simulink library "correlator_library"  (Simulink 6.2)
undefined symbols (not defined in the file or in its folder): BitWidthIn, BramDepth, phase_swtich_counter_width
libraries: xbsIndex_r3 x200, correlator_library x31, fft_library x11
(part 2 of 2)

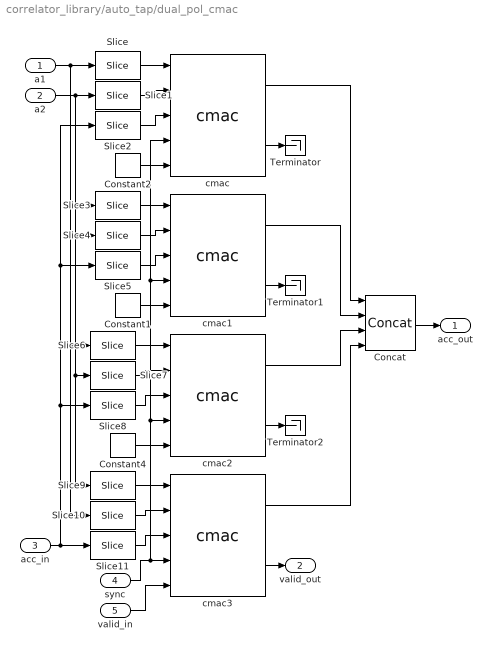
== system correlator_library/auto_tap/dual_pol_cmac ==
  a1 : Inport  Port=1  LatchInput=off
  a2 : Inport  Port=2  LatchInput=off
  acc_in : Inport  Port=3  LatchInput=off
  sync : Inport  Port=4  LatchInput=off
  valid_in : Inport  Port=5  LatchInput=off
  Concat : xbsIndex_r3/Concat  num_inputs=4  explicit_period=off  period=1  dbl_ovrd=off
  Constant1 : xbsIndex_r3/Constant  const=0  arith_type=Unsigned  n_bits=1  bin_pt=0  explicit_period=off  period=1  dbl_ovrd=off
  Constant2 : xbsIndex_r3/Constant  const=0  arith_type=Unsigned  n_bits=1  bin_pt=0  explicit_period=off  period=1  dbl_ovrd=off
  Constant4 : xbsIndex_r3/Constant  const=0  arith_type=Unsigned  n_bits=1  bin_pt=0  explicit_period=off  period=1  dbl_ovrd=off
  Slice{,1,6,9} (4 alike) : xbsIndex_r3/Slice  mode=Upper Bit Location + Width  nbits=2*BitWidthIn  bit1=0  base1=MSB of Input  bit0=0  base0=LSB of Input  boolean_output=off  explicit_period=off  period=1  dbl_ovrd=off
  Slice{3..4,7,10} (4 alike) : xbsIndex_r3/Slice  mode=Upper Bit Location + Width  nbits=2*BitWidthIn  bit1=-2*BitWidthIn  base1=MSB of Input  bit0=0  base0=LSB of Input  boolean_output=off  explicit_period=off  period=1  dbl_ovrd=off
  Slice11 : xbsIndex_r3/Slice  mode=Upper Bit Location + Width  nbits=2*BitWidthOut  bit1=-6*BitWidthOut  base1=MSB of Input  bit0=0  base0=LSB of Input  boolean_output=off  explicit_period=off  period=1  dbl_ovrd=off
  Slice2 : xbsIndex_r3/Slice  mode=Upper Bit Location + Width  nbits=2*BitWidthOut  bit1=0  base1=MSB of Input  bit0=0  base0=LSB of Input  boolean_output=off  explicit_period=off  period=1  dbl_ovrd=off
  Slice5 : xbsIndex_r3/Slice  mode=Upper Bit Location + Width  nbits=2*BitWidthOut  bit1=-2*BitWidthOut  base1=MSB of Input  bit0=0  base0=LSB of Input  boolean_output=off  explicit_period=off  period=1  dbl_ovrd=off
  Slice8 : xbsIndex_r3/Slice  mode=Upper Bit Location + Width  nbits=2*BitWidthOut  bit1=-4*BitWidthOut  base1=MSB of Input  bit0=0  base0=LSB of Input  boolean_output=off  explicit_period=off  period=1  dbl_ovrd=off
  Terminator : Terminator
  Terminator1 : Terminator
  Terminator2 : Terminator
  cmac{,1..3} (4 alike) : correlator_library/cmac  BitWidthIn=BitWidthIn  BitWidthOut=BitWidthOut  AccLen=AccLen  MultLatency=MultLatency  AddLatency=AddLatency  use_conj=on  use_mult_core=off
  acc_out : Outport
  valid_out : Outport  Port=2
  wires:
  Slice/1 -> cmac/1
  Slice1/1 -> cmac/2
  Slice2/1 -> cmac/3
  Slice3/1 -> cmac1/1
  Slice4/1 -> cmac1/2
  Slice5/1 -> cmac1/3
  Concat/1 -> acc_out/1
  Constant2/1 -> cmac/5
  cmac/2 -> Terminator/1
  Constant1/1 -> cmac1/5
  Slice6/1 -> cmac2/1
  Slice7/1 -> cmac2/2
  Slice8/1 -> cmac2/3
  Constant4/1 -> cmac2/5
  Slice9/1 -> cmac3/1
  Slice10/1 -> cmac3/2
  Slice11/1 -> cmac3/3
  valid_in/1 -> cmac3/5
  sync/1 -> cmac3/4, cmac2/4, cmac1/4, cmac/4
  cmac1/2 -> Terminator1/1
  cmac2/2 -> Terminator2/1
  cmac3/2 -> valid_out/1
  cmac/1 -> Concat/1
  cmac1/1 -> Concat/2
  cmac2/1 -> Concat/3
  cmac3/1 -> Concat/4
  a1/1 -> Slice/1, Slice3/1, Slice6/1, Slice10/1
  a2/1 -> Slice1/1, Slice4/1, Slice7/1, Slice9/1
  acc_in/1 -> Slice11/1, Slice8/1, Slice5/1, Slice2/1

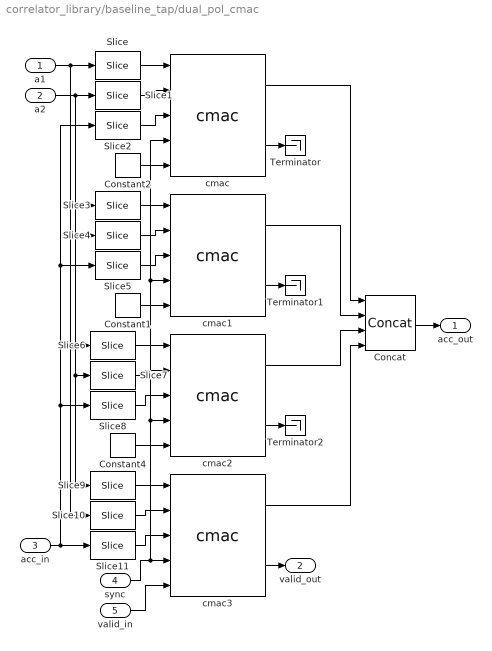
== system correlator_library/baseline_tap/dual_pol_cmac ==
  a1 : Inport  Port=1  LatchInput=off
  a2 : Inport  Port=2  LatchInput=off
  acc_in : Inport  Port=3  LatchInput=off
  sync : Inport  Port=4  LatchInput=off
  valid_in : Inport  Port=5  LatchInput=off
  Concat : xbsIndex_r3/Concat  num_inputs=4  explicit_period=off  period=1  dbl_ovrd=off
  Constant1 : xbsIndex_r3/Constant  const=0  arith_type=Unsigned  n_bits=1  bin_pt=0  explicit_period=off  period=1  dbl_ovrd=off
  Constant2 : xbsIndex_r3/Constant  const=0  arith_type=Unsigned  n_bits=1  bin_pt=0  explicit_period=off  period=1  dbl_ovrd=off
  Constant4 : xbsIndex_r3/Constant  const=0  arith_type=Unsigned  n_bits=1  bin_pt=0  explicit_period=off  period=1  dbl_ovrd=off
  Slice{,1,6,9} (4 alike) : xbsIndex_r3/Slice  mode=Upper Bit Location + Width  nbits=2*BitWidthIn  bit1=0  base1=MSB of Input  bit0=0  base0=LSB of Input  boolean_output=off  explicit_period=off  period=1  dbl_ovrd=off
  Slice{3..4,7,10} (4 alike) : xbsIndex_r3/Slice  mode=Upper Bit Location + Width  nbits=2*BitWidthIn  bit1=-2*BitWidthIn  base1=MSB of Input  bit0=0  base0=LSB of Input  boolean_output=off  explicit_period=off  period=1  dbl_ovrd=off
  Slice11 : xbsIndex_r3/Slice  mode=Upper Bit Location + Width  nbits=2*BitWidthOut  bit1=-6*BitWidthOut  base1=MSB of Input  bit0=0  base0=LSB of Input  boolean_output=off  explicit_period=off  period=1  dbl_ovrd=off
  Slice2 : xbsIndex_r3/Slice  mode=Upper Bit Location + Width  nbits=2*BitWidthOut  bit1=0  base1=MSB of Input  bit0=0  base0=LSB of Input  boolean_output=off  explicit_period=off  period=1  dbl_ovrd=off
  Slice5 : xbsIndex_r3/Slice  mode=Upper Bit Location + Width  nbits=2*BitWidthOut  bit1=-2*BitWidthOut  base1=MSB of Input  bit0=0  base0=LSB of Input  boolean_output=off  explicit_period=off  period=1  dbl_ovrd=off
  Slice8 : xbsIndex_r3/Slice  mode=Upper Bit Location + Width  nbits=2*BitWidthOut  bit1=-4*BitWidthOut  base1=MSB of Input  bit0=0  base0=LSB of Input  boolean_output=off  explicit_period=off  period=1  dbl_ovrd=off
  Terminator : Terminator
  Terminator1 : Terminator
  Terminator2 : Terminator
  cmac{,1..3} (4 alike) : correlator_library/cmac  BitWidthIn=BitWidthIn  BitWidthOut=BitWidthOut  AccLen=AccLen  MultLatency=MultLatency  AddLatency=AddLatency  use_conj=on  use_mult_core=off
  acc_out : Outport
  valid_out : Outport  Port=2
  wires:
  acc_in/1 -> Slice2/1, Slice5/1, Slice8/1, Slice11/1
  a2/1 -> Slice9/1, Slice7/1, Slice4/1, Slice1/1
  a1/1 -> Slice10/1, Slice6/1, Slice3/1, Slice/1
  cmac3/1 -> Concat/4
  cmac2/1 -> Concat/3
  cmac1/1 -> Concat/2
  cmac/1 -> Concat/1
  cmac3/2 -> valid_out/1
  cmac2/2 -> Terminator2/1
  cmac1/2 -> Terminator1/1
  sync/1 -> cmac/4, cmac1/4, cmac2/4, cmac3/4
  valid_in/1 -> cmac3/5
  Slice11/1 -> cmac3/3
  Slice10/1 -> cmac3/2
  Slice9/1 -> cmac3/1
  Constant4/1 -> cmac2/5
  Slice8/1 -> cmac2/3
  Slice7/1 -> cmac2/2
  Slice6/1 -> cmac2/1
  Constant1/1 -> cmac1/5
  cmac/2 -> Terminator/1
  Constant2/1 -> cmac/5
  Concat/1 -> acc_out/1
  Slice5/1 -> cmac1/3
  Slice4/1 -> cmac1/2
  Slice3/1 -> cmac1/1
  Slice2/1 -> cmac/3
  Slice1/1 -> cmac/2
  Slice/1 -> cmac/1

== system correlator_library/cm/cm ==
  a : Inport  Port=1  LatchInput=off
  b : Inport  Port=2  LatchInput=off
  c : Inport  Port=3  LatchInput=off
  d : Inport  Port=4  LatchInput=off
  ac : xbsIndex_r3/Mult  precision=Full  arith_type="Signed  (2's comp)"  n_bits=8  bin_pt=2  quantization=Truncate  overflow=Wrap  latency=mult_latency  explicit_period=off  period=1  en=off  dbl_ovrd=off  show_param=off  mult_type=Parallel  oversample=2  use_embedded=on  pipeline=on  use_rpm=on  placement_style=Rectangular Shape  gen_core=off
      settings: xl_area=[0, 0, 0, 0, 0, 0, 0]
  ad : xbsIndex_r3/Mult  precision=Full  arith_type="Signed  (2's comp)"  n_bits=8  bin_pt=2  quantization=Truncate  overflow=Wrap  latency=mult_latency  explicit_period=off  period=1  en=off  dbl_ovrd=off  show_param=off  mult_type=Parallel  oversample=2  use_embedded=on  pipeline=on  use_rpm=on  placement_style=Rectangular Shape  gen_core=off
      settings: xl_area=[0, 0, 0, 0, 0, 0, 0]
  bc : xbsIndex_r3/Mult  precision=Full  arith_type="Signed  (2's comp)"  n_bits=8  bin_pt=2  quantization=Truncate  overflow=Wrap  latency=mult_latency  explicit_period=off  period=1  en=off  dbl_ovrd=off  show_param=off  mult_type=Parallel  oversample=2  use_embedded=on  pipeline=on  use_rpm=on  placement_style=Rectangular Shape  gen_core=off
      settings: xl_area=[0, 0, 0, 0, 0, 0, 0]
  bd : xbsIndex_r3/Mult  precision=Full  arith_type="Signed  (2's comp)"  n_bits=8  bin_pt=2  quantization=Truncate  overflow=Wrap  latency=mult_latency  explicit_period=off  period=1  en=off  dbl_ovrd=off  show_param=off  mult_type=Parallel  oversample=2  use_embedded=on  pipeline=on  use_rpm=on  placement_style=Rectangular Shape  gen_core=off
      settings: xl_area=[0, 0, 0, 0, 0, 0, 0]
  imag_sum : xbsIndex_r3/AddSub  mode=Subtraction  precision=User Defined  arith_type=Unsigned  n_bits=n_bits  bin_pt=bin_pt  quantization="Round  (unbiased: +/- Inf)"  overflow=Wrap  latency=add_latency  explicit_period=off  period=1  use_carryin=off  use_carryout=off  en=off  dbl_ovrd=off  show_param=off  use_core=on  pipeline=off  use_rpm=on  gen_core=off
      settings: xl_area=[0, 0, 0, 0, 0, 0, 0]
  real_sum : xbsIndex_r3/AddSub  mode=Addition  precision=User Defined  arith_type=Unsigned  n_bits=n_bits  bin_pt=bin_pt  quantization="Round  (unbiased: +/- Inf)"  overflow=Wrap  latency=add_latency  explicit_period=off  period=1  use_carryin=off  use_carryout=off  en=off  dbl_ovrd=off  show_param=off  use_core=on  pipeline=off  use_rpm=on  gen_core=off
      settings: xl_area=[0, 0, 0, 0, 0, 0, 0]
  real : Outport
  imag : Outport  Port=2
  wires:
  imag_sum/1 -> imag/1
  real_sum/1 -> real/1
  d/1 -> bd/2, ad/2
  b/1 -> bd/1, bc/1
  c/1 -> ac/2, bc/2
  a/1 -> ac/1, ad/1
  ad/1 -> imag_sum/2
  bc/1 -> imag_sum/1
  bd/1 -> real_sum/2
  ac/1 -> real_sum/1

== system correlator_library/x_engine/auto_tap ==
  a_del : Inport  Port=1  LatchInput=off
  a_ndel : Inport  Port=2  LatchInput=off
  a_loop : Inport  Port=3  LatchInput=off
  a_end : Inport  Port=4  LatchInput=off
  acc_in : Inport  Port=5  LatchInput=off
  valid_in : Inport  Port=6  LatchInput=off
  sync_in : Inport  Port=7  LatchInput=off
  Delay6 : xbsIndex_r3/Delay  latency=1  reg_retiming=off  explicit_period=off  period=1  en=off  accept_only_valid=off  init_zero=on  dbl_ovrd=off  show_param=off
      settings: xl_area=[0, 0, 0, 0, 0, 0, 0]
  dual_pol_cmac : Subsystem  mask{BitWidthIn=BitWidthIn, BitWidthOut=BitWidthOut, AccLen=AccLen, MultLatency=MultLatency, AddLatency=AddLatency, use_mult_core=off}
      mask prompts: BitWidthIn "Bit Width of Sample In"; BitWidthOut "Bit Width of Sample Out"; AccLen "Accumulation Length"; MultLatency "Mult Latency"; AddLatency "Add Latency"; use_mult_core "Use Dedicated Multipliers"
      mask init: same as correlator_library/auto_tap/dual_pol_cmac
  a_del_out : Outport
  a_ndel_out : Outport  Port=2
  a_loop_out : Outport  Port=3
  a_end_out : Outport  Port=4
  acc_out : Outport  Port=5
  valid_out : Outport  Port=6
  rst_out : Outport  Port=7
  sync_out : Outport  Port=8
  wires:
  Delay6/1 -> dual_pol_cmac/4(sync)
  sync_in/1 -> sync_out/1, Delay6/1, rst_out/1
  a_del/1 -> dual_pol_cmac/1(a1), a_del_out/1
  dual_pol_cmac/1(acc_out) -> acc_out/1
  acc_in/1 -> dual_pol_cmac/3(acc_in)
  dual_pol_cmac/2(valid_out) -> valid_out/1
  valid_in/1 -> dual_pol_cmac/5(valid_in)
  a_ndel/1 -> dual_pol_cmac/2(a2), a_ndel_out/1
  a_end/1 -> a_end_out/1
  a_loop/1 -> a_loop_out/1

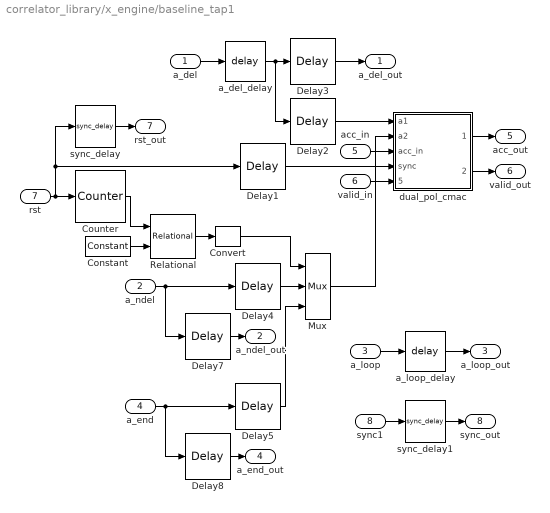
== system correlator_library/x_engine/baseline_tap1 ==
  a_del : Inport  Port=1  LatchInput=off
  a_ndel : Inport  Port=2  LatchInput=off
  a_loop : Inport  Port=3  LatchInput=off
  a_end : Inport  Port=4  LatchInput=off
  acc_in : Inport  Port=5  LatchInput=off
  valid_in : Inport  Port=6  LatchInput=off
  rst : Inport  Port=7  LatchInput=off
  sync1 : Inport  Port=8  LatchInput=off
  Constant : xbsIndex_r3/Constant  const=(AntNum - AntSep) * AccLen  equ=P=C  arith_type=Unsigned  n_bits=AntBits + BitGrowth  bin_pt=0  opselect=C  inp2=PCIN>>17  opr=+  inp1=P  carry=CIN  iostate=0  explicit_period=off  period=1  dbl_ovrd=off
  Convert : xbsIndex_r3/Convert  arith_type=Unsigned  n_bits=1  bin_pt=0  quantization=Truncate  overflow=Wrap  latency=0  explicit_period=off  period=1  dbl_ovrd=off  show_param=off  inserted_by_tool=off  pipeline=off
      settings: xl_area=[0, 0, 0, 0, 0, 0, 0]
  Counter : xbsIndex_r3/Counter  cnt_type=Count Limited  n_bits=AntBits + BitGrowth  bin_pt=0  arith_type=Unsigned  start_count=0  cnt_to=AntNum * AccLen - 1  cnt_by_val=1  operation=Up  explicit_period=off  period=1  load_pin=off  rst=on  en=off  dbl_ovrd=off  show_param=off  use_rpm=on  gen_core=off
      settings: xl_area=[0, 0, 0, 0, 0, 0, 0]
  Delay1 : xbsIndex_r3/Delay  latency=2  reg_retiming=off  explicit_period=off  period=1  en=off  accept_only_valid=off  init_zero=on  dbl_ovrd=off  show_param=off
      settings: xl_area=[0, 0, 0, 0, 0, 0, 0]
  Delay2 : xbsIndex_r3/Delay  latency=2  reg_retiming=off  explicit_period=off  period=1  en=off  accept_only_valid=off  init_zero=on  dbl_ovrd=off  show_param=off
      settings: xl_area=[0, 0, 0, 0, 0, 0, 0]
  Delay3 : xbsIndex_r3/Delay  latency=1  reg_retiming=off  explicit_period=off  period=1  en=off  accept_only_valid=off  init_zero=on  dbl_ovrd=off  show_param=off
      settings: xl_area=[0, 0, 0, 0, 0, 0, 0]
  Delay{4..5,7..8} (4 alike) : xbsIndex_r3/Delay  latency=1  reg_retiming=off  explicit_period=on  period=1  en=off  accept_only_valid=off  init_zero=on  dbl_ovrd=off  show_param=off
      settings: xl_area=[0, 0, 0, 0, 0, 0, 0]
  Mux : xbsIndex_r3/Mux  inputs=2  precision=Full  arith_type="Signed  (2's comp)"  n_bits=8  bin_pt=2  quantization=Truncate  overflow=Wrap  latency=1  explicit_period=off  period=1  en=off  dbl_ovrd=off  show_param=off  mux_type=off  use_rpm=off  gen_core=off
      settings: xl_area=[0, 0, 0, 0, 0, 0, 0]
  Relational : xbsIndex_r3/Relational  mode=a>=b  latency=1  explicit_period=off  period=1  en=off  dbl_ovrd=off  show_param=off
      settings: xl_area=[0, 0, 0, 0, 0, 0, 0]
  a_del_delay : fft_library/delay  DelayLen=AccLen
  a_loop_delay : fft_library/delay  DelayLen=AccLen - 1
  dual_pol_cmac : Subsystem  mask{BitWidthIn=BitWidthIn, BitWidthOut=BitWidthOut, AccLen=AccLen, MultLatency=MultLatency, AddLatency=AddLatency, use_mult_core=off}
      mask prompts: BitWidthIn "Bit Width of Sample In"; BitWidthOut "Bit Width of Sample Out"; AccLen "Accumulation Length"; MultLatency "Mult Latency"; AddLatency "Add Latency"; use_mult_core "Use Dedicated Multipliers"
      mask init: same as correlator_library/auto_tap/dual_pol_cmac
  sync_delay : fft_library/sync_delay  DelayLen=AccLen + 1
  sync_delay1 : fft_library/sync_delay  DelayLen=2 * AccLen
  a_del_out : Outport
  a_ndel_out : Outport  Port=2
  a_loop_out : Outport  Port=3
  a_end_out : Outport  Port=4
  acc_out : Outport  Port=5
  valid_out : Outport  Port=6
  rst_out : Outport  Port=7
  sync_out : Outport  Port=8
  wires:
  sync1/1 -> sync_delay1/1
  sync_delay1/1 -> sync_out/1
  sync_delay/1 -> rst_out/1
  Delay8/1 -> a_end_out/1
  Delay7/1 -> a_ndel_out/1
  Delay3/1 -> a_del_out/1
  a_loop_delay/1 -> a_loop_out/1
  a_loop/1 -> a_loop_delay/1
  a_end/1 -> Delay8/1, Delay5/1
  a_ndel/1 -> Delay7/1, Delay4/1
  valid_in/1 -> dual_pol_cmac/5(valid_in)
  dual_pol_cmac/2(valid_out) -> valid_out/1
  acc_in/1 -> dual_pol_cmac/3(acc_in)
  dual_pol_cmac/1(acc_out) -> acc_out/1
  a_del/1 -> a_del_delay/1
  rst/1 -> sync_delay/1, Delay1/1, Counter/1
  Delay1/1 -> dual_pol_cmac/4(sync)
  Convert/1 -> Mux/1
  Relational/1 -> Convert/1
  Constant/1 -> Relational/2
  Counter/1 -> Relational/1
  Mux/1 -> dual_pol_cmac/2(a2)
  Delay2/1 -> dual_pol_cmac/1(a1)
  a_del_delay/1 -> Delay3/1, Delay2/1
  Delay5/1 -> Mux/3
  Delay4/1 -> Mux/2

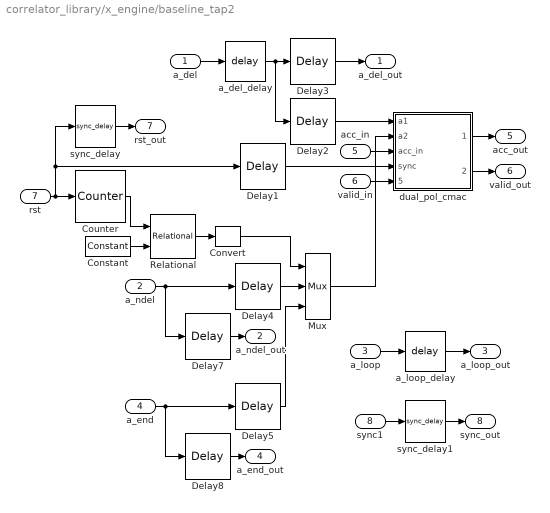
== system correlator_library/x_engine/baseline_tap2 ==
  a_del : Inport  Port=1  LatchInput=off
  a_ndel : Inport  Port=2  LatchInput=off
  a_loop : Inport  Port=3  LatchInput=off
  a_end : Inport  Port=4  LatchInput=off
  acc_in : Inport  Port=5  LatchInput=off
  valid_in : Inport  Port=6  LatchInput=off
  rst : Inport  Port=7  LatchInput=off
  sync1 : Inport  Port=8  LatchInput=off
  Constant : xbsIndex_r3/Constant  const=(AntNum - AntSep) * AccLen  equ=P=C  arith_type=Unsigned  n_bits=AntBits + BitGrowth  bin_pt=0  opselect=C  inp2=PCIN>>17  opr=+  inp1=P  carry=CIN  iostate=0  explicit_period=off  period=1  dbl_ovrd=off
  Convert : xbsIndex_r3/Convert  arith_type=Unsigned  n_bits=1  bin_pt=0  quantization=Truncate  overflow=Wrap  latency=0  explicit_period=off  period=1  dbl_ovrd=off  show_param=off  inserted_by_tool=off  pipeline=off
      settings: xl_area=[0, 0, 0, 0, 0, 0, 0]
  Counter : xbsIndex_r3/Counter  cnt_type=Count Limited  n_bits=AntBits + BitGrowth  bin_pt=0  arith_type=Unsigned  start_count=0  cnt_to=AntNum * AccLen - 1  cnt_by_val=1  operation=Up  explicit_period=off  period=1  load_pin=off  rst=on  en=off  dbl_ovrd=off  show_param=off  use_rpm=on  gen_core=off
      settings: xl_area=[0, 0, 0, 0, 0, 0, 0]
  Delay1 : xbsIndex_r3/Delay  latency=2  reg_retiming=off  explicit_period=off  period=1  en=off  accept_only_valid=off  init_zero=on  dbl_ovrd=off  show_param=off
      settings: xl_area=[0, 0, 0, 0, 0, 0, 0]
  Delay2 : xbsIndex_r3/Delay  latency=2  reg_retiming=off  explicit_period=off  period=1  en=off  accept_only_valid=off  init_zero=on  dbl_ovrd=off  show_param=off
      settings: xl_area=[0, 0, 0, 0, 0, 0, 0]
  Delay3 : xbsIndex_r3/Delay  latency=1  reg_retiming=off  explicit_period=off  period=1  en=off  accept_only_valid=off  init_zero=on  dbl_ovrd=off  show_param=off
      settings: xl_area=[0, 0, 0, 0, 0, 0, 0]
  Delay{4..5,7..8} (4 alike) : xbsIndex_r3/Delay  latency=1  reg_retiming=off  explicit_period=on  period=1  en=off  accept_only_valid=off  init_zero=on  dbl_ovrd=off  show_param=off
      settings: xl_area=[0, 0, 0, 0, 0, 0, 0]
  Mux : xbsIndex_r3/Mux  inputs=2  precision=Full  arith_type="Signed  (2's comp)"  n_bits=8  bin_pt=2  quantization=Truncate  overflow=Wrap  latency=1  explicit_period=off  period=1  en=off  dbl_ovrd=off  show_param=off  mux_type=off  use_rpm=off  gen_core=off
      settings: xl_area=[0, 0, 0, 0, 0, 0, 0]
  Relational : xbsIndex_r3/Relational  mode=a>=b  latency=1  explicit_period=off  period=1  en=off  dbl_ovrd=off  show_param=off
      settings: xl_area=[0, 0, 0, 0, 0, 0, 0]
  a_del_delay : fft_library/delay  DelayLen=AccLen
  a_loop_delay : fft_library/delay  DelayLen=AccLen - 1
  dual_pol_cmac : Subsystem  mask{BitWidthIn=BitWidthIn, BitWidthOut=BitWidthOut, AccLen=AccLen, MultLatency=MultLatency, AddLatency=AddLatency, use_mult_core=off}
      mask prompts: BitWidthIn "Bit Width of Sample In"; BitWidthOut "Bit Width of Sample Out"; AccLen "Accumulation Length"; MultLatency "Mult Latency"; AddLatency "Add Latency"; use_mult_core "Use Dedicated Multipliers"
      mask init: same as correlator_library/auto_tap/dual_pol_cmac
  sync_delay : fft_library/sync_delay  DelayLen=AccLen + 1
  sync_delay1 : fft_library/sync_delay  DelayLen=2 * AccLen
  a_del_out : Outport
  a_ndel_out : Outport  Port=2
  a_loop_out : Outport  Port=3
  a_end_out : Outport  Port=4
  acc_out : Outport  Port=5
  valid_out : Outport  Port=6
  rst_out : Outport  Port=7
  sync_out : Outport  Port=8
  wires:
  sync1/1 -> sync_delay1/1
  sync_delay1/1 -> sync_out/1
  sync_delay/1 -> rst_out/1
  Delay8/1 -> a_end_out/1
  Delay7/1 -> a_ndel_out/1
  Delay3/1 -> a_del_out/1
  a_loop_delay/1 -> a_loop_out/1
  a_loop/1 -> a_loop_delay/1
  a_end/1 -> Delay8/1, Delay5/1
  a_ndel/1 -> Delay7/1, Delay4/1
  valid_in/1 -> dual_pol_cmac/5(valid_in)
  dual_pol_cmac/2(valid_out) -> valid_out/1
  acc_in/1 -> dual_pol_cmac/3(acc_in)
  dual_pol_cmac/1(acc_out) -> acc_out/1
  a_del/1 -> a_del_delay/1
  rst/1 -> sync_delay/1, Delay1/1, Counter/1
  Delay1/1 -> dual_pol_cmac/4(sync)
  Convert/1 -> Mux/1
  Relational/1 -> Convert/1
  Constant/1 -> Relational/2
  Counter/1 -> Relational/1
  Mux/1 -> dual_pol_cmac/2(a2)
  Delay2/1 -> dual_pol_cmac/1(a1)
  a_del_delay/1 -> Delay3/1, Delay2/1
  Delay5/1 -> Mux/3
  Delay4/1 -> Mux/2

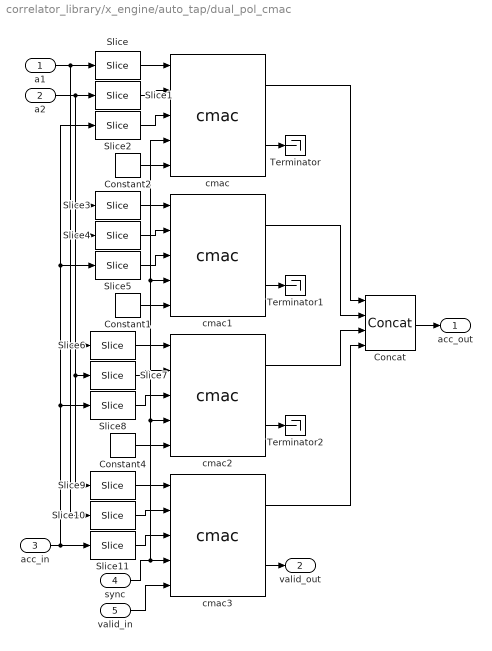
== system correlator_library/x_engine/auto_tap/dual_pol_cmac ==
  a1 : Inport  Port=1  LatchInput=off
  a2 : Inport  Port=2  LatchInput=off
  acc_in : Inport  Port=3  LatchInput=off
  sync : Inport  Port=4  LatchInput=off
  valid_in : Inport  Port=5  LatchInput=off
  Concat : xbsIndex_r3/Concat  num_inputs=4  explicit_period=off  period=1  dbl_ovrd=off
  Constant1 : xbsIndex_r3/Constant  const=0  arith_type=Unsigned  n_bits=1  bin_pt=0  explicit_period=off  period=1  dbl_ovrd=off
  Constant2 : xbsIndex_r3/Constant  const=0  arith_type=Unsigned  n_bits=1  bin_pt=0  explicit_period=off  period=1  dbl_ovrd=off
  Constant4 : xbsIndex_r3/Constant  const=0  arith_type=Unsigned  n_bits=1  bin_pt=0  explicit_period=off  period=1  dbl_ovrd=off
  Slice{,1,6,9} (4 alike) : xbsIndex_r3/Slice  mode=Upper Bit Location + Width  nbits=2*BitWidthIn  bit1=0  base1=MSB of Input  bit0=0  base0=LSB of Input  boolean_output=off  explicit_period=off  period=1  dbl_ovrd=off
  Slice{3..4,7,10} (4 alike) : xbsIndex_r3/Slice  mode=Upper Bit Location + Width  nbits=2*BitWidthIn  bit1=-2*BitWidthIn  base1=MSB of Input  bit0=0  base0=LSB of Input  boolean_output=off  explicit_period=off  period=1  dbl_ovrd=off
  Slice11 : xbsIndex_r3/Slice  mode=Upper Bit Location + Width  nbits=2*BitWidthOut  bit1=-6*BitWidthOut  base1=MSB of Input  bit0=0  base0=LSB of Input  boolean_output=off  explicit_period=off  period=1  dbl_ovrd=off
  Slice2 : xbsIndex_r3/Slice  mode=Upper Bit Location + Width  nbits=2*BitWidthOut  bit1=0  base1=MSB of Input  bit0=0  base0=LSB of Input  boolean_output=off  explicit_period=off  period=1  dbl_ovrd=off
  Slice5 : xbsIndex_r3/Slice  mode=Upper Bit Location + Width  nbits=2*BitWidthOut  bit1=-2*BitWidthOut  base1=MSB of Input  bit0=0  base0=LSB of Input  boolean_output=off  explicit_period=off  period=1  dbl_ovrd=off
  Slice8 : xbsIndex_r3/Slice  mode=Upper Bit Location + Width  nbits=2*BitWidthOut  bit1=-4*BitWidthOut  base1=MSB of Input  bit0=0  base0=LSB of Input  boolean_output=off  explicit_period=off  period=1  dbl_ovrd=off
  Terminator : Terminator
  Terminator1 : Terminator
  Terminator2 : Terminator
  cmac{,1..3} (4 alike) : correlator_library/cmac  BitWidthIn=BitWidthIn  BitWidthOut=BitWidthOut  AccLen=AccLen  MultLatency=MultLatency  AddLatency=AddLatency  use_conj=on  use_mult_core=off
  acc_out : Outport
  valid_out : Outport  Port=2
  wires:
  acc_in/1 -> Slice2/1, Slice5/1, Slice8/1, Slice11/1
  a2/1 -> Slice9/1, Slice7/1, Slice4/1, Slice1/1
  a1/1 -> Slice10/1, Slice6/1, Slice3/1, Slice/1
  cmac3/1 -> Concat/4
  cmac2/1 -> Concat/3
  cmac1/1 -> Concat/2
  cmac/1 -> Concat/1
  cmac3/2 -> valid_out/1
  cmac2/2 -> Terminator2/1
  cmac1/2 -> Terminator1/1
  sync/1 -> cmac/4, cmac1/4, cmac2/4, cmac3/4
  valid_in/1 -> cmac3/5
  Slice11/1 -> cmac3/3
  Slice10/1 -> cmac3/2
  Slice9/1 -> cmac3/1
  Constant4/1 -> cmac2/5
  Slice8/1 -> cmac2/3
  Slice7/1 -> cmac2/2
  Slice6/1 -> cmac2/1
  Constant1/1 -> cmac1/5
  cmac/2 -> Terminator/1
  Constant2/1 -> cmac/5
  Concat/1 -> acc_out/1
  Slice5/1 -> cmac1/3
  Slice4/1 -> cmac1/2
  Slice3/1 -> cmac1/1
  Slice2/1 -> cmac/3
  Slice1/1 -> cmac/2
  Slice/1 -> cmac/1

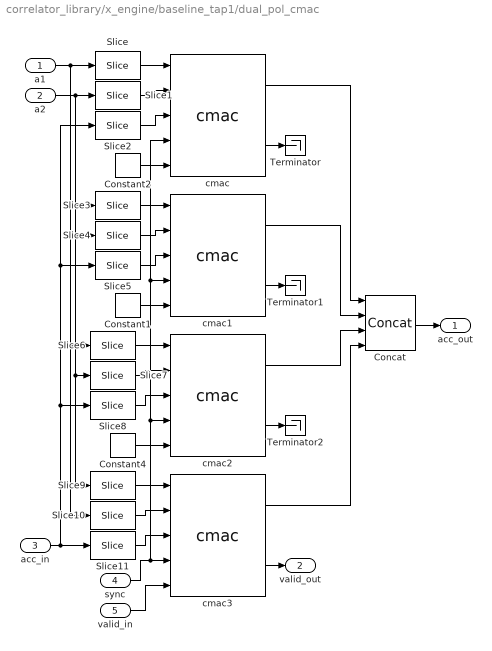
== system correlator_library/x_engine/baseline_tap1/dual_pol_cmac ==
  a1 : Inport  Port=1  LatchInput=off
  a2 : Inport  Port=2  LatchInput=off
  acc_in : Inport  Port=3  LatchInput=off
  sync : Inport  Port=4  LatchInput=off
  valid_in : Inport  Port=5  LatchInput=off
  Concat : xbsIndex_r3/Concat  num_inputs=4  explicit_period=off  period=1  dbl_ovrd=off
  Constant1 : xbsIndex_r3/Constant  const=0  arith_type=Unsigned  n_bits=1  bin_pt=0  explicit_period=off  period=1  dbl_ovrd=off
  Constant2 : xbsIndex_r3/Constant  const=0  arith_type=Unsigned  n_bits=1  bin_pt=0  explicit_period=off  period=1  dbl_ovrd=off
  Constant4 : xbsIndex_r3/Constant  const=0  arith_type=Unsigned  n_bits=1  bin_pt=0  explicit_period=off  period=1  dbl_ovrd=off
  Slice{,1,6,9} (4 alike) : xbsIndex_r3/Slice  mode=Upper Bit Location + Width  nbits=2*BitWidthIn  bit1=0  base1=MSB of Input  bit0=0  base0=LSB of Input  boolean_output=off  explicit_period=off  period=1  dbl_ovrd=off
  Slice{3..4,7,10} (4 alike) : xbsIndex_r3/Slice  mode=Upper Bit Location + Width  nbits=2*BitWidthIn  bit1=-2*BitWidthIn  base1=MSB of Input  bit0=0  base0=LSB of Input  boolean_output=off  explicit_period=off  period=1  dbl_ovrd=off
  Slice11 : xbsIndex_r3/Slice  mode=Upper Bit Location + Width  nbits=2*BitWidthOut  bit1=-6*BitWidthOut  base1=MSB of Input  bit0=0  base0=LSB of Input  boolean_output=off  explicit_period=off  period=1  dbl_ovrd=off
  Slice2 : xbsIndex_r3/Slice  mode=Upper Bit Location + Width  nbits=2*BitWidthOut  bit1=0  base1=MSB of Input  bit0=0  base0=LSB of Input  boolean_output=off  explicit_period=off  period=1  dbl_ovrd=off
  Slice5 : xbsIndex_r3/Slice  mode=Upper Bit Location + Width  nbits=2*BitWidthOut  bit1=-2*BitWidthOut  base1=MSB of Input  bit0=0  base0=LSB of Input  boolean_output=off  explicit_period=off  period=1  dbl_ovrd=off
  Slice8 : xbsIndex_r3/Slice  mode=Upper Bit Location + Width  nbits=2*BitWidthOut  bit1=-4*BitWidthOut  base1=MSB of Input  bit0=0  base0=LSB of Input  boolean_output=off  explicit_period=off  period=1  dbl_ovrd=off
  Terminator : Terminator
  Terminator1 : Terminator
  Terminator2 : Terminator
  cmac{,1..3} (4 alike) : correlator_library/cmac  BitWidthIn=BitWidthIn  BitWidthOut=BitWidthOut  AccLen=AccLen  MultLatency=MultLatency  AddLatency=AddLatency  use_conj=on  use_mult_core=off
  acc_out : Outport
  valid_out : Outport  Port=2
  wires:
  Slice/1 -> cmac/1
  Slice1/1 -> cmac/2
  Slice2/1 -> cmac/3
  Slice3/1 -> cmac1/1
  Slice4/1 -> cmac1/2
  Slice5/1 -> cmac1/3
  Concat/1 -> acc_out/1
  Constant2/1 -> cmac/5
  cmac/2 -> Terminator/1
  Constant1/1 -> cmac1/5
  Slice6/1 -> cmac2/1
  Slice7/1 -> cmac2/2
  Slice8/1 -> cmac2/3
  Constant4/1 -> cmac2/5
  Slice9/1 -> cmac3/1
  Slice10/1 -> cmac3/2
  Slice11/1 -> cmac3/3
  valid_in/1 -> cmac3/5
  sync/1 -> cmac3/4, cmac2/4, cmac1/4, cmac/4
  cmac1/2 -> Terminator1/1
  cmac2/2 -> Terminator2/1
  cmac3/2 -> valid_out/1
  cmac/1 -> Concat/1
  cmac1/1 -> Concat/2
  cmac2/1 -> Concat/3
  cmac3/1 -> Concat/4
  a1/1 -> Slice/1, Slice3/1, Slice6/1, Slice10/1
  a2/1 -> Slice1/1, Slice4/1, Slice7/1, Slice9/1
  acc_in/1 -> Slice11/1, Slice8/1, Slice5/1, Slice2/1

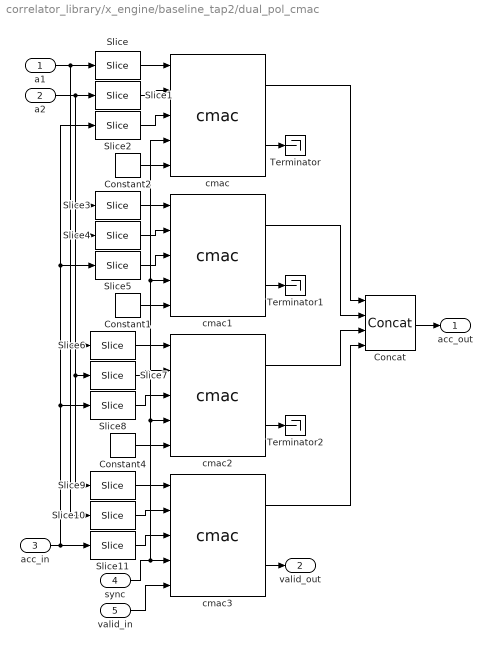
== system correlator_library/x_engine/baseline_tap2/dual_pol_cmac ==
  a1 : Inport  Port=1  LatchInput=off
  a2 : Inport  Port=2  LatchInput=off
  acc_in : Inport  Port=3  LatchInput=off
  sync : Inport  Port=4  LatchInput=off
  valid_in : Inport  Port=5  LatchInput=off
  Concat : xbsIndex_r3/Concat  num_inputs=4  explicit_period=off  period=1  dbl_ovrd=off
  Constant1 : xbsIndex_r3/Constant  const=0  arith_type=Unsigned  n_bits=1  bin_pt=0  explicit_period=off  period=1  dbl_ovrd=off
  Constant2 : xbsIndex_r3/Constant  const=0  arith_type=Unsigned  n_bits=1  bin_pt=0  explicit_period=off  period=1  dbl_ovrd=off
  Constant4 : xbsIndex_r3/Constant  const=0  arith_type=Unsigned  n_bits=1  bin_pt=0  explicit_period=off  period=1  dbl_ovrd=off
  Slice{,1,6,9} (4 alike) : xbsIndex_r3/Slice  mode=Upper Bit Location + Width  nbits=2*BitWidthIn  bit1=0  base1=MSB of Input  bit0=0  base0=LSB of Input  boolean_output=off  explicit_period=off  period=1  dbl_ovrd=off
  Slice{3..4,7,10} (4 alike) : xbsIndex_r3/Slice  mode=Upper Bit Location + Width  nbits=2*BitWidthIn  bit1=-2*BitWidthIn  base1=MSB of Input  bit0=0  base0=LSB of Input  boolean_output=off  explicit_period=off  period=1  dbl_ovrd=off
  Slice11 : xbsIndex_r3/Slice  mode=Upper Bit Location + Width  nbits=2*BitWidthOut  bit1=-6*BitWidthOut  base1=MSB of Input  bit0=0  base0=LSB of Input  boolean_output=off  explicit_period=off  period=1  dbl_ovrd=off
  Slice2 : xbsIndex_r3/Slice  mode=Upper Bit Location + Width  nbits=2*BitWidthOut  bit1=0  base1=MSB of Input  bit0=0  base0=LSB of Input  boolean_output=off  explicit_period=off  period=1  dbl_ovrd=off
  Slice5 : xbsIndex_r3/Slice  mode=Upper Bit Location + Width  nbits=2*BitWidthOut  bit1=-2*BitWidthOut  base1=MSB of Input  bit0=0  base0=LSB of Input  boolean_output=off  explicit_period=off  period=1  dbl_ovrd=off
  Slice8 : xbsIndex_r3/Slice  mode=Upper Bit Location + Width  nbits=2*BitWidthOut  bit1=-4*BitWidthOut  base1=MSB of Input  bit0=0  base0=LSB of Input  boolean_output=off  explicit_period=off  period=1  dbl_ovrd=off
  Terminator : Terminator
  Terminator1 : Terminator
  Terminator2 : Terminator
  cmac{,1..3} (4 alike) : correlator_library/cmac  BitWidthIn=BitWidthIn  BitWidthOut=BitWidthOut  AccLen=AccLen  MultLatency=MultLatency  AddLatency=AddLatency  use_conj=on  use_mult_core=off
  acc_out : Outport
  valid_out : Outport  Port=2
  wires:
  Slice/1 -> cmac/1
  Slice1/1 -> cmac/2
  Slice2/1 -> cmac/3
  Slice3/1 -> cmac1/1
  Slice4/1 -> cmac1/2
  Slice5/1 -> cmac1/3
  Concat/1 -> acc_out/1
  Constant2/1 -> cmac/5
  cmac/2 -> Terminator/1
  Constant1/1 -> cmac1/5
  Slice6/1 -> cmac2/1
  Slice7/1 -> cmac2/2
  Slice8/1 -> cmac2/3
  Constant4/1 -> cmac2/5
  Slice9/1 -> cmac3/1
  Slice10/1 -> cmac3/2
  Slice11/1 -> cmac3/3
  valid_in/1 -> cmac3/5
  sync/1 -> cmac3/4, cmac2/4, cmac1/4, cmac/4
  cmac1/2 -> Terminator1/1
  cmac2/2 -> Terminator2/1
  cmac3/2 -> valid_out/1
  cmac/1 -> Concat/1
  cmac1/1 -> Concat/2
  cmac2/1 -> Concat/3
  cmac3/1 -> Concat/4
  a1/1 -> Slice/1, Slice3/1, Slice6/1, Slice10/1
  a2/1 -> Slice1/1, Slice4/1, Slice7/1, Slice9/1
  acc_in/1 -> Slice11/1, Slice8/1, Slice5/1, Slice2/1
